simulink library "aircraft_lib"  (Simulink 7.2)
settings: Solver=ode45  SolverMode=SingleTasking  StartTime=0.0  StopTime=10.0  RelTol=1e-3
undefined symbols (not defined in the file or in its folder): runway_alt
libraries: acparams_lib x2, actuator_T2_lib x2, aero_lib x2, auxvars_lib x2, avionics_T2_lib x2, eomlib x2, engine_T2_lib x2, gravity_lib x2, landinggear_lib x2, sensors_T2_lib x2, aircraft_lib x1, simulink x1
settings Model: Creator=Austin Murch  LastModifiedBy=E183308  ExtModeAutoUpdateStatusClock=off

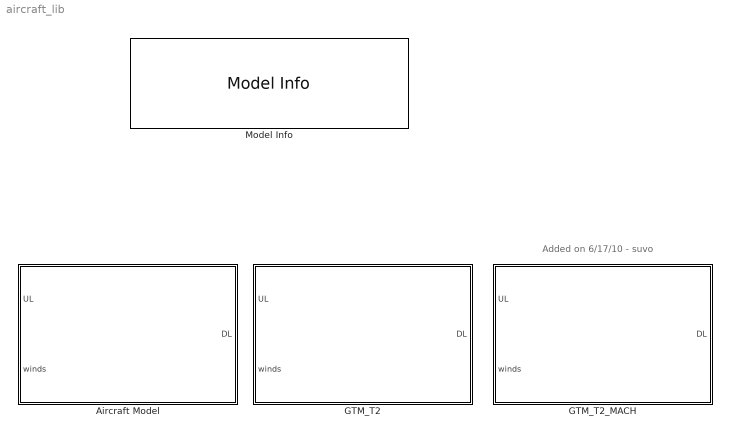
== system aircraft_lib ==
  note: Added on 6/17/10 - suvo
  Aircraft Model : Subsystem  BlockChoice=GTM_T2
      settings: TemplateBlock=self  MemberBlocks=GTM_T2,GTM_T2_MACH
  GTM_T2 : Subsystem  Tag=From trunk/GTMsim/gtm_model.mdl revision 162
      mask Display: image(imread('GTMtiny.png'))
  GTM_T2_MACH : Subsystem  Tag=From trunk/GTMsim/gtm_model.mdl revision 162
      mask Display: image(imread('GTMtiny.png'))
  Model Info : simulink/Model-Wide Utilities/Model Info  SystemSampleTime=-1  InitialBlockCM=None  BlockCM=None  Frame=on  DisplayStringWithTags=|  HorizontalTextAlignment=Center  LeftAlignmentValue=0.5  SourceBlockDiagram=aircraft_lib  TagMaxNumber=20
      | Aircraft Plant Library
      | %<ModelVersion>
      | Las modified by %<LastModifiedBy> on %<LastModificationDate>

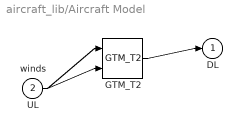
== system aircraft_lib/Aircraft Model ==
  UL : Inport  OutDataType=sfix(16)  OutScaling=2^0
  winds : Inport  Port=2  OutDataType=sfix(16)  OutScaling=2^0
  GTM_T2 : aircraft_lib/GTM_T2  Tag=From trunk/GTMsim/gtm_model.mdl revision 162  SystemSampleTime=-1
  DL : Outport  OutDataType=sfix(16)  OutScaling=2^0
  wires:
  UL/1 -> GTM_T2/1
  winds/1 -> GTM_T2/2
  GTM_T2/1 -> DL/1

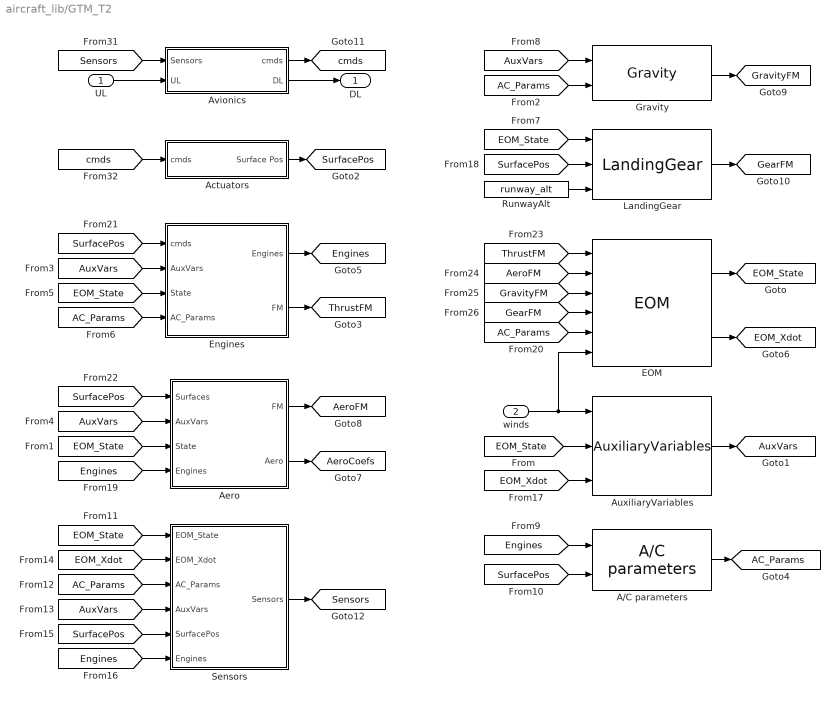
== system aircraft_lib/GTM_T2 ==
  UL : Inport  OutDataType=sfix(16)  OutScaling=2^0
  winds : Inport  Port=2  PortDimensions=6  OutDataType=sfix(16)  OutScaling=2^0
  A/C parameters : acparams_lib/A//C parameters  SystemSampleTime=-1
  Actuators : Subsystem  BlockChoice=GTM_T2
      settings: AttributesFormatString=%<BlockChoice>  TemplateBlock=actuator_lib/Actuators  MemberBlocks=GTM_T2
  Aero : Subsystem  BlockChoice=GTM_T2
      settings: AttributesFormatString=%<BlockChoice>  TemplateBlock=aero_lib/Aero  MemberBlocks=GTM_T2
  AuxiliaryVariables : auxvars_lib/AuxiliaryVariables  SystemSampleTime=-1
  Avionics : Subsystem  BlockChoice=GTM_T2
      settings: AttributesFormatString=%<BlockChoice>  TemplateBlock=avionics_lib/Avionics  MemberBlocks=Blank,GTM_T2
  EOM : eomlib/EOM  SystemSampleTime=-1
  Engines : Subsystem  BlockChoice=GTM_T2
      link override GTM_T2/Left_Engine: BlockChoice=Jetcat P70
      link override GTM_T2/Right_Engine: BlockChoice=Jetcat P70
      settings: AttributesFormatString=%<BlockChoice>  TemplateBlock=enginelib/Engines  MemberBlocks=GTM_T2
  Gravity : gravity_lib/Gravity  SystemSampleTime=-1
  LandingGear : landinggear_lib/LandingGear  SystemSampleTime=-1  GEAR_SPRING=25*12  zeta=0.4  NoseWheelRate=0.15
  RunwayAlt : Constant  Value=runway_alt  OutDataType=sfix(16)  OutScaling=2^0
  Sensors : Subsystem  BlockChoice=GTM_T2
      settings: AttributesFormatString=%<BlockChoice>  TemplateBlock=sensors_lib/Sensors  MemberBlocks=Blank,GTM_T2,GTM_T2 gtm_design
  DL : Outport  OutDataType=sfix(16)  OutScaling=2^0
  tag scope: AC_Params=global, AeroCoefs=global, AeroFM=global, AuxVars=global, EOM_State=global, EOM_Xdot=global, Engines=global, GearFM=global, GravityFM=global, Sensors=global, SurfacePos=global, ThrustFM=global, cmds=global
  wires:
  UL/1 -> Avionics/2(UL)
  Avionics/2(DL) -> DL/1
  Gravity/1 -> [GravityFM]
  [AuxVars] -> Sensors/4(AuxVars)
  [EOM_Xdot] -> Sensors/2(EOM_Xdot)
  [Engines] -> Sensors/6(Engines)
  [SurfacePos] -> Sensors/5(SurfacePos)
  [AC_Params] -> Sensors/3(AC_Params)
  [EOM_State] -> Sensors/1(EOM_State)
  [AC_Params] -> EOM/5
  [GearFM] -> EOM/4
  [GravityFM] -> EOM/3
  [AeroFM] -> EOM/2
  [ThrustFM] -> EOM/1
  [EOM_State] -> AuxiliaryVariables/2
  Aero/2(Aero) -> [AeroCoefs]
  [SurfacePos] -> Aero/1(Surfaces)
  RunwayAlt/1 -> LandingGear/3
  [SurfacePos] -> Engines/1(cmds)
  EOM/2 -> [EOM_Xdot]
  [Engines] -> Aero/4(Engines)
  [EOM_Xdot] -> AuxiliaryVariables/3
  Engines/1(Engines) -> [Engines]
  [SurfacePos] -> A/C parameters/2
  [Engines] -> A/C parameters/1
  A/C parameters/1 -> [AC_Params]
  [AC_Params] -> Engines/4(AC_Params)
  [AuxVars] -> Engines/2(AuxVars)
  [EOM_State] -> Engines/3(State)
  [AuxVars] -> Gravity/1
  [AC_Params] -> Gravity/2
  EOM/1 -> [EOM_State]
  Engines/2(FM) -> [ThrustFM]
  Aero/1(FM) -> [AeroFM]
  [AuxVars] -> Aero/2(AuxVars)
  AuxiliaryVariables/1 -> [AuxVars]
  [EOM_State] -> Aero/3(State)
  [EOM_State] -> LandingGear/1
  [SurfacePos] -> LandingGear/2
  LandingGear/1 -> [GearFM]
  Actuators/1(Surface Pos) -> [SurfacePos]
  winds/1 -> AuxiliaryVariables/1, EOM/6
  Avionics/1(cmds) -> [cmds]
  [Sensors] -> Avionics/1(Sensors)
  [cmds] -> Actuators/1(cmds)
  Sensors/1(Sensors) -> [Sensors]

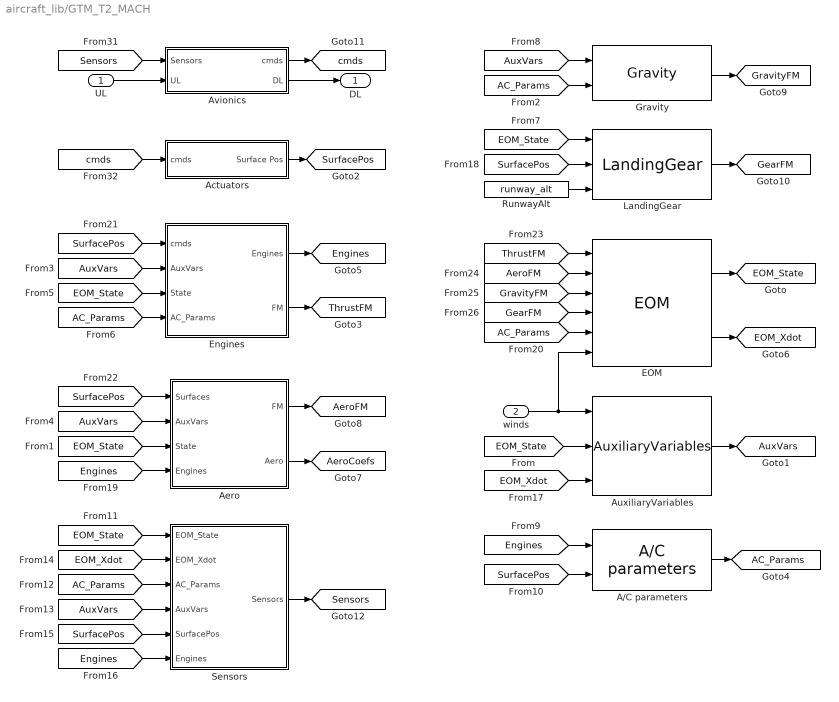
== system aircraft_lib/GTM_T2_MACH ==
  UL : Inport  OutDataType=sfix(16)  OutScaling=2^0
  winds : Inport  Port=2  PortDimensions=6  OutDataType=sfix(16)  OutScaling=2^0
  A/C parameters : acparams_lib/A//C parameters  SystemSampleTime=-1
  Actuators : Subsystem  BlockChoice=GTM_T2
      settings: AttributesFormatString=%<BlockChoice>  TemplateBlock=actuator_lib/Actuators  MemberBlocks=GTM_T2
  Aero : Subsystem  BlockChoice=GTM_T2
      settings: AttributesFormatString=%<BlockChoice>  TemplateBlock=aero_lib/Aero  MemberBlocks=GTM_T2
  AuxiliaryVariables : auxvars_lib/AuxiliaryVariables  SystemSampleTime=-1
  Avionics : Subsystem  BlockChoice=GTM_T2
      settings: AttributesFormatString=%<BlockChoice>  TemplateBlock=avionics_lib/Avionics  MemberBlocks=Blank,GTM_T2,TransportDelay
  EOM : eomlib/EOM  SystemSampleTime=-1
  Engines : Subsystem  BlockChoice=GTM_T2_MACH
      link override GTM_T2/Left_Engine: BlockChoice=Jetcat P70
      link override GTM_T2/Right_Engine: BlockChoice=Jetcat P70
      settings: AttributesFormatString=%<BlockChoice>  TemplateBlock=enginelib/Engines  MemberBlocks=GTM_T2,GTM_T2_MACH
  Gravity : gravity_lib/Gravity  SystemSampleTime=-1
  LandingGear : landinggear_lib/LandingGear  SystemSampleTime=-1  GEAR_SPRING=25*12  zeta=0.4  NoseWheelRate=0.15
  RunwayAlt : Constant  Value=runway_alt  OutDataType=sfix(16)  OutScaling=2^0
  Sensors : Subsystem  BlockChoice=GTM_T2
      settings: AttributesFormatString=%<BlockChoice>  TemplateBlock=sensors_lib/Sensors  MemberBlocks=Blank,GTM_T2,GTM_T2 gtm_design
  DL : Outport  OutDataType=sfix(16)  OutScaling=2^0
  tag scope: AC_Params=global, AeroCoefs=global, AeroFM=global, AuxVars=global, EOM_State=global, EOM_Xdot=global, Engines=global, GearFM=global, GravityFM=global, Sensors=global, SurfacePos=global, ThrustFM=global, cmds=global
  wires:
  Sensors/1(Sensors) -> [Sensors]
  [cmds] -> Actuators/1(cmds)
  [Sensors] -> Avionics/1(Sensors)
  Avionics/1(cmds) -> [cmds]
  winds/1 -> EOM/6, AuxiliaryVariables/1
  Actuators/1(Surface Pos) -> [SurfacePos]
  LandingGear/1 -> [GearFM]
  [SurfacePos] -> LandingGear/2
  [EOM_State] -> LandingGear/1
  [EOM_State] -> Aero/3(State)
  AuxiliaryVariables/1 -> [AuxVars]
  [AuxVars] -> Aero/2(AuxVars)
  Aero/1(FM) -> [AeroFM]
  Engines/2(FM) -> [ThrustFM]
  EOM/1 -> [EOM_State]
  [AC_Params] -> Gravity/2
  [AuxVars] -> Gravity/1
  [EOM_State] -> Engines/3(State)
  [AuxVars] -> Engines/2(AuxVars)
  [AC_Params] -> Engines/4(AC_Params)
  A/C parameters/1 -> [AC_Params]
  [Engines] -> A/C parameters/1
  [SurfacePos] -> A/C parameters/2
  Engines/1(Engines) -> [Engines]
  [EOM_Xdot] -> AuxiliaryVariables/3
  [Engines] -> Aero/4(Engines)
  EOM/2 -> [EOM_Xdot]
  [SurfacePos] -> Engines/1(cmds)
  RunwayAlt/1 -> LandingGear/3
  [SurfacePos] -> Aero/1(Surfaces)
  Aero/2(Aero) -> [AeroCoefs]
  [EOM_State] -> AuxiliaryVariables/2
  [ThrustFM] -> EOM/1
  [AeroFM] -> EOM/2
  [GravityFM] -> EOM/3
  [GearFM] -> EOM/4
  [AC_Params] -> EOM/5
  [EOM_State] -> Sensors/1(EOM_State)
  [AC_Params] -> Sensors/3(AC_Params)
  [SurfacePos] -> Sensors/5(SurfacePos)
  [Engines] -> Sensors/6(Engines)
  [EOM_Xdot] -> Sensors/2(EOM_Xdot)
  [AuxVars] -> Sensors/4(AuxVars)
  Gravity/1 -> [GravityFM]
  Avionics/2(DL) -> DL/1
  UL/1 -> Avionics/2(UL)

== system aircraft_lib/GTM_T2/Actuators ==
  cmds : Inport  OutDataType=sfix(16)  OutScaling=2^0
  GTM_T2 : actuator_T2_lib/GTM_T2  SystemSampleTime=-1
  Surface Pos : Outport  OutDataType=sfix(16)  OutScaling=2^0
  wires:
  cmds/1 -> GTM_T2/1
  GTM_T2/1 -> Surface Pos/1

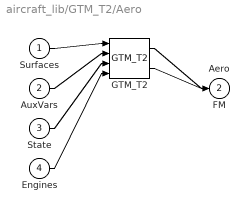
== system aircraft_lib/GTM_T2/Aero ==
  Surfaces : Inport  OutDataType=sfix(16)  OutScaling=2^0
  AuxVars : Inport  Port=2  OutDataType=sfix(16)  OutScaling=2^0
  State : Inport  Port=3  OutDataType=sfix(16)  OutScaling=2^0
  Engines : Inport  Port=4  OutDataType=sfix(16)  OutScaling=2^0
  GTM_T2 : aero_lib/GTM_T2  SystemSampleTime=-1
  FM : Outport  OutDataType=sfix(16)  OutScaling=2^0
  Aero : Outport  Port=2  OutDataType=sfix(16)  OutScaling=2^0
  wires:
  Surfaces/1 -> GTM_T2/1
  AuxVars/1 -> GTM_T2/2
  State/1 -> GTM_T2/3
  Engines/1 -> GTM_T2/4
  GTM_T2/1 -> FM/1
  GTM_T2/2 -> Aero/1

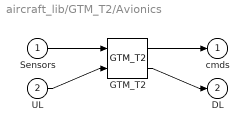
== system aircraft_lib/GTM_T2/Avionics ==
  Sensors : Inport  OutDataType=sfix(16)  OutScaling=2^0
  UL : Inport  Port=2  OutDataType=sfix(16)  OutScaling=2^0
  GTM_T2 : avionics_T2_lib/GTM_T2  SystemSampleTime=-1
  cmds : Outport  OutDataType=sfix(16)  OutScaling=2^0
  DL : Outport  Port=2  OutDataType=sfix(16)  OutScaling=2^0
  wires:
  Sensors/1 -> GTM_T2/1
  UL/1 -> GTM_T2/2
  GTM_T2/1 -> cmds/1
  GTM_T2/2 -> DL/1

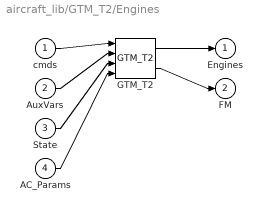
== system aircraft_lib/GTM_T2/Engines ==
  cmds : Inport  OutDataType=sfix(16)  OutScaling=2^0
  AuxVars : Inport  Port=2  OutDataType=sfix(16)  OutScaling=2^0
  State : Inport  Port=3  OutDataType=sfix(16)  OutScaling=2^0
  AC_Params : Inport  Port=4  OutDataType=sfix(16)  OutScaling=2^0
  GTM_T2 : engine_T2_lib/GTM_T2  SystemSampleTime=-1
  Engines : Outport  OutDataType=sfix(16)  OutScaling=2^0
  FM : Outport  Port=2  OutDataType=sfix(16)  OutScaling=2^0
  wires:
  cmds/1 -> GTM_T2/1
  AuxVars/1 -> GTM_T2/2
  State/1 -> GTM_T2/3
  AC_Params/1 -> GTM_T2/4
  GTM_T2/1 -> Engines/1
  GTM_T2/2 -> FM/1

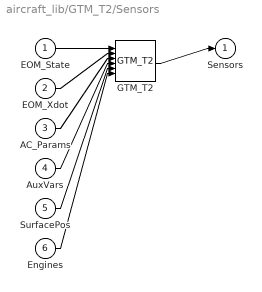
== system aircraft_lib/GTM_T2/Sensors ==
  EOM_State : Inport  OutDataType=sfix(16)  OutScaling=2^0
  EOM_Xdot : Inport  Port=2  OutDataType=sfix(16)  OutScaling=2^0
  AC_Params : Inport  Port=3  OutDataType=sfix(16)  OutScaling=2^0
  AuxVars : Inport  Port=4  OutDataType=sfix(16)  OutScaling=2^0
  SurfacePos : Inport  Port=5  OutDataType=sfix(16)  OutScaling=2^0
  Engines : Inport  Port=6  OutDataType=sfix(16)  OutScaling=2^0
  GTM_T2 : sensors_T2_lib/GTM_T2  SystemSampleTime=-1
  Sensors : Outport  OutDataType=sfix(16)  OutScaling=2^0
  wires:
  EOM_State/1 -> GTM_T2/1
  EOM_Xdot/1 -> GTM_T2/2
  AC_Params/1 -> GTM_T2/3
  AuxVars/1 -> GTM_T2/4
  SurfacePos/1 -> GTM_T2/5
  Engines/1 -> GTM_T2/6
  GTM_T2/1 -> Sensors/1

== system aircraft_lib/GTM_T2_MACH/Actuators ==
  cmds : Inport  OutDataType=sfix(16)  OutScaling=2^0
  GTM_T2 : actuator_T2_lib/GTM_T2  SystemSampleTime=-1
  Surface Pos : Outport  OutDataType=sfix(16)  OutScaling=2^0
  wires:
  cmds/1 -> GTM_T2/1
  GTM_T2/1 -> Surface Pos/1

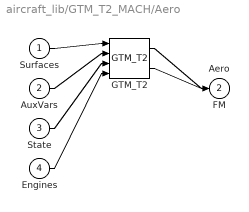
== system aircraft_lib/GTM_T2_MACH/Aero ==
  Surfaces : Inport  OutDataType=sfix(16)  OutScaling=2^0
  AuxVars : Inport  Port=2  OutDataType=sfix(16)  OutScaling=2^0
  State : Inport  Port=3  OutDataType=sfix(16)  OutScaling=2^0
  Engines : Inport  Port=4  OutDataType=sfix(16)  OutScaling=2^0
  GTM_T2 : aero_lib/GTM_T2  SystemSampleTime=-1
  FM : Outport  OutDataType=sfix(16)  OutScaling=2^0
  Aero : Outport  Port=2  OutDataType=sfix(16)  OutScaling=2^0
  wires:
  Surfaces/1 -> GTM_T2/1
  AuxVars/1 -> GTM_T2/2
  State/1 -> GTM_T2/3
  Engines/1 -> GTM_T2/4
  GTM_T2/1 -> FM/1
  GTM_T2/2 -> Aero/1

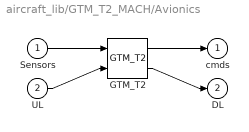
== system aircraft_lib/GTM_T2_MACH/Avionics ==
  Sensors : Inport  OutDataType=sfix(16)  OutScaling=2^0
  UL : Inport  Port=2  OutDataType=sfix(16)  OutScaling=2^0
  GTM_T2 : avionics_T2_lib/GTM_T2  SystemSampleTime=-1
  cmds : Outport  OutDataType=sfix(16)  OutScaling=2^0
  DL : Outport  Port=2  OutDataType=sfix(16)  OutScaling=2^0
  wires:
  Sensors/1 -> GTM_T2/1
  UL/1 -> GTM_T2/2
  GTM_T2/1 -> cmds/1
  GTM_T2/2 -> DL/1

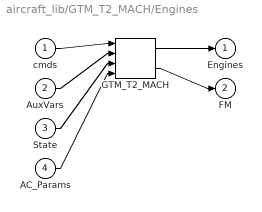
== system aircraft_lib/GTM_T2_MACH/Engines ==
  cmds : Inport  OutDataType=sfix(16)  OutScaling=2^0
  AuxVars : Inport  Port=2  OutDataType=sfix(16)  OutScaling=2^0
  State : Inport  Port=3  OutDataType=sfix(16)  OutScaling=2^0
  AC_Params : Inport  Port=4  OutDataType=sfix(16)  OutScaling=2^0
  GTM_T2_MACH : engine_T2_lib/GTM_T2_MACH  SystemSampleTime=-1
  Engines : Outport  OutDataType=sfix(16)  OutScaling=2^0
  FM : Outport  Port=2  OutDataType=sfix(16)  OutScaling=2^0
  wires:
  cmds/1 -> GTM_T2_MACH/1
  AuxVars/1 -> GTM_T2_MACH/2
  State/1 -> GTM_T2_MACH/3
  AC_Params/1 -> GTM_T2_MACH/4
  GTM_T2_MACH/1 -> Engines/1
  GTM_T2_MACH/2 -> FM/1

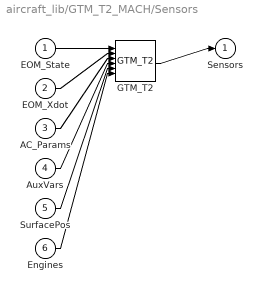
== system aircraft_lib/GTM_T2_MACH/Sensors ==
  EOM_State : Inport  OutDataType=sfix(16)  OutScaling=2^0
  EOM_Xdot : Inport  Port=2  OutDataType=sfix(16)  OutScaling=2^0
  AC_Params : Inport  Port=3  OutDataType=sfix(16)  OutScaling=2^0
  AuxVars : Inport  Port=4  OutDataType=sfix(16)  OutScaling=2^0
  SurfacePos : Inport  Port=5  OutDataType=sfix(16)  OutScaling=2^0
  Engines : Inport  Port=6  OutDataType=sfix(16)  OutScaling=2^0
  GTM_T2 : sensors_T2_lib/GTM_T2  SystemSampleTime=-1
  Sensors : Outport  OutDataType=sfix(16)  OutScaling=2^0
  wires:
  EOM_State/1 -> GTM_T2/1
  EOM_Xdot/1 -> GTM_T2/2
  AC_Params/1 -> GTM_T2/3
  AuxVars/1 -> GTM_T2/4
  SurfacePos/1 -> GTM_T2/5
  Engines/1 -> GTM_T2/6
  GTM_T2/1 -> Sensors/1
